simulink model "3"  (R2021a)
settings: Solver=FixedStepDiscrete  StartTime=0.0  StopTime=inf  FixedStep=0.1  RelTol=1e-3  EnableMultiTasking=on
settings Model: Creator=smrh1  LastModifiedBy=smrh1
settings SolverCC: AlgebraicLoopSolver=TrustRegion  AutoInsertRateTranBlk=on
settings OptimizationCC: LifeSpan=inf
settings DebuggingCC: SFUnexpectedBacktrackingDiag=warning  SFNoUnconditionalDefaultTransitionDiag=warning  SFExecutionAtInitializationDiag=none  ArithmeticOperatorsInVariantConditions=warning
settings SFSimCC: SimUseLocalCustomCode=off  CustomCodeUndefinedFunction=UseInterfaceOnly
settings RTWCC: RTWUseLocalCustomCode=off
settings CodeAppCC: StateflowObjectComments=on
settings GRTTargetCC: TargetLangStandard=C89/C90 (ANSI)
settings ConfigComp: CovMetricSettings=dw  CovSaveCumulativeToWorkspaceVar=on  CovSaveSingleToWorkspaceVar=on  CovExternalEMLEnable=off

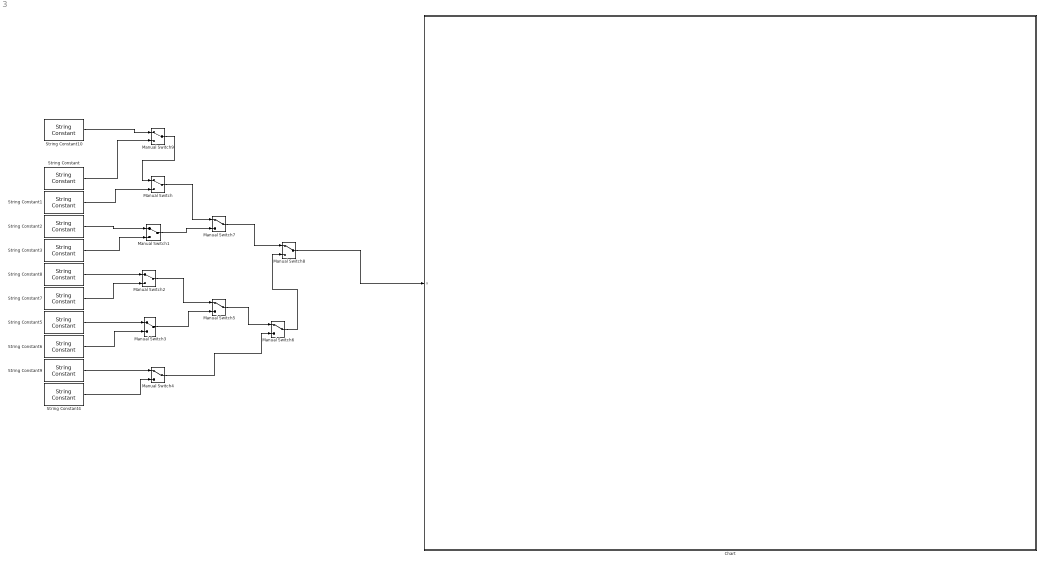
== system 3 ==
  Chart : Stateflow chart  TreatAsAtomicUnit=on
  Manual Switch{,1..9} (10 alike) : ManualSwitch
  String Constant : StringConstant  String="\"f\""
  String Constant1 : StringConstant  String="\"c\""
  String Constant10 : StringConstant  String="\"\""
  String Constant2 : StringConstant  String="\"b\""
  String Constant3 : StringConstant  String="\"b\""
  String Constant4 : StringConstant  String="\"f\""
  String Constant5 : StringConstant  String="\"d\""
  String Constant6 : StringConstant  String="\"a\""
  String Constant7 : StringConstant  String="\"b\""
  String Constant8 : StringConstant  String="\"f\""
  String Constant9 : StringConstant  String="\"e\""
  wires:
  String Constant1/1 -> Manual Switch/2
  String Constant2/1 -> Manual Switch1/1
  String Constant3/1 -> Manual Switch1/2
  String Constant8/1 -> Manual Switch2/1
  String Constant7/1 -> Manual Switch2/2
  String Constant5/1 -> Manual Switch3/1
  String Constant9/1 -> Manual Switch4/1
  String Constant4/1 -> Manual Switch4/2
  Manual Switch/1 -> Manual Switch7/1
  Manual Switch1/1 -> Manual Switch7/2
  Manual Switch2/1 -> Manual Switch5/1
  Manual Switch3/1 -> Manual Switch5/2
  Manual Switch5/1 -> Manual Switch6/1
  Manual Switch4/1 -> Manual Switch6/2
  Manual Switch7/1 -> Manual Switch8/1
  Manual Switch6/1 -> Manual Switch8/2
  Manual Switch8/1 -> Chart/1(x)
  String Constant6/1 -> Manual Switch3/2
  String Constant/1 -> Manual Switch9/2
  String Constant10/1 -> Manual Switch9/1
  Manual Switch9/1 -> Manual Switch/1

== stateflow chart 3/Chart ==
  state state2
    state state6
      state d [parallel]
        settings: executionOrder=3
        state state8
        state state9
        state9 -> state8 : [x=="a" & hasChanged(x)]
        state8 -> state9 : [x=="b"& hasChanged(x)]
        (default) -> state9
      state e [parallel]
        settings: executionOrder=1
        state state10
        state state11
        state11 -> state10 : [x=="c"& hasChanged(x)]
        state10 -> state11 : [x=="c"& hasChanged(x)]
        (default) -> state11
      state f [parallel]
        settings: executionOrder=2
        state state12
        state state13
        f -> f
        state13 -> state12 : [x=="c"& hasChanged(x)]
        state12 -> state13 : [x=="a"& hasChanged(x)]
        (default) -> state13
    state state7
    state7 -> state6 [order 2] : [x=="e"& hasChanged(x)]
    state6 -> state7 : [x=="d"& hasChanged(x)]
    (default) -> state6
  state state1
    (history)
    state state4
    state state5
    (default) -> state4
    state5 -> state4 : [x=="a"& hasChanged(x)]
    state4 -> state5 : [x=="b"& hasChanged(x)]
  state state3
  (default) -> state1
  state1 -> state2 [order 1] : [x=="f" & hasChanged(x)]
  state3 -> state5 : [x=="e"& hasChanged(x)]
  state7 -> state1 [order 1] : [x=="b"& hasChanged(x)]
  state1 -> state3 [order 2] : [x=="d"& hasChanged(x)]
  data: x input string
